simulink model "Motor_Position"  (R2020b)
settings: Solver=VariableStepAuto  StartTime=0.0  StopTime=0.2  RelTol=1e-3
values from neighbouring files (symbols this model uses):
  b = 3.5077E-6    [Problem4.sldd]    (also in Problem4_params.m = 3.5077e-06)
  J = 3.2284E-6    [Problem4.sldd]    (also in Problem4_params.m = 3.2284e-06)
  K = 0.0274    [Problem4.sldd]    (also in Problem4_params.m)
  L = 2.75E-6    [Problem4.sldd]    (also in Problem4_params.m = 2.75e-06)
  R = 4.0    [Problem4.sldd]    (also in Problem4_params.m = 4)
settings Model: DataDictionary=Problem4.sldd  Creator=Shirish  LastModifiedBy=Shirish
settings DataIOCC: SaveOutput=off  SaveTime=off

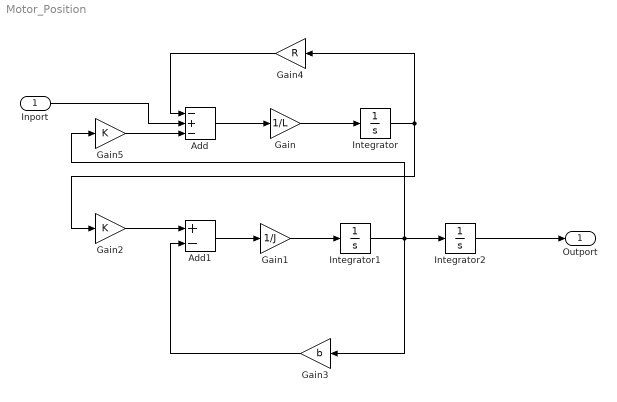
== system Motor_Position ==
  Inport : Inport  OutDataTypeStr=double  PortDimensions=1  SampleTime=0
  Add : Sum  Inputs=-+-
  Add1 : Sum  Inputs=+-
  Gain : Gain  Gain=1/L
  Gain1 : Gain  Gain=1/J
  Gain2 : Gain  Gain=K
  Gain3 : Gain  Gain=b
  Gain4 : Gain  Gain=R
  Gain5 : Gain  Gain=K
  Integrator : Integrator
  Integrator1 : Integrator
  Integrator2 : Integrator
  Outport : Outport  OutDataTypeStr=double  PortDimensions=1  SampleTime=0
  wires:
  Gain2/1 -> Add1/1
  Gain5/1 -> Add/3
  Integrator1/1 -> Integrator2/1, Gain3/1, Gain5/1
  Gain3/1 -> Add1/2
  Integrator/1 -> Gain2/1, Gain4/1
  Integrator2/1 -> Outport/1
  Add/1 -> Gain/1
  Inport/1 -> Add/2
  Gain4/1 -> Add/1
  Gain1/1 -> Integrator1/1
  Add1/1 -> Gain1/1
  Gain/1 -> Integrator/1
